simulink model "ThrusterModel0"  (R2018b)
settings: configuration reference "RPi_ControlRate" (kept outside this file)
InitFcn:
  | loadThrusterData
settings Model: Creator=Andy  LastModifiedBy=barthal
settings ConfigSetRef: SourceLocation=Base Workspace

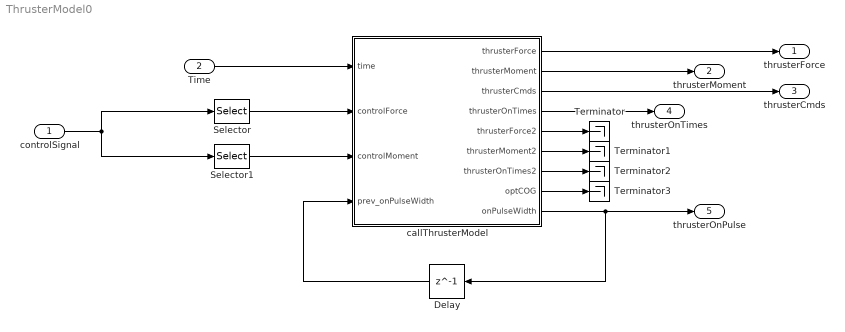
== system ThrusterModel0 ==
  controlSignal : Inport  OutDataTypeStr=double
  Time : Inport  Port=2  OutDataTypeStr=double  PortDimensions=1
  Delay : Delay  DelayLength=1  InitialCondition=[0 0 0 0 0 0 0 0]
  Selector : Selector  InputPortWidth=6  IndexOptions=Index vector (dialog)  Indices=[1 2 3]  OutputSizes=1
  Selector1 : Selector  InputPortWidth=6  IndexOptions=Index vector (dialog)  Indices=[4:6]  OutputSizes=1
  Terminator{,1..3} (4 alike) : Terminator
  callThrusterModel : MATLAB Function  TreatAsAtomicUnit=on
  thrusterForce : Outport  OutDataTypeStr=double
  thrusterMoment : Outport  Port=2  OutDataTypeStr=double
  thrusterCmds : Outport  Port=3  OutDataTypeStr=boolean
  thrusterOnTimes : Outport  Port=4
  thrusterOnPulse : Outport  Port=5
  wires:
  Time/1 -> callThrusterModel/1(time)
  controlSignal/1 -> Selector1/1, Selector/1
  callThrusterModel/4(thrusterOnTimes) -> thrusterOnTimes/1
  callThrusterModel/1(thrusterForce) -> thrusterForce/1
  callThrusterModel/2(thrusterMoment) -> thrusterMoment/1
  Selector/1 -> callThrusterModel/2(controlForce)
  Selector1/1 -> callThrusterModel/3(controlMoment)
  callThrusterModel/3(thrusterCmds) -> thrusterCmds/1
  callThrusterModel/9(onPulseWidth) -> thrusterOnPulse/1, Delay/1
  Delay/1 -> callThrusterModel/4(prev_onPulseWidth)
  callThrusterModel/5(thrusterForce2) -> Terminator/1
  callThrusterModel/6(thrusterMoment2) -> Terminator1/1
  callThrusterModel/7(thrusterOnTimes2) -> Terminator2/1
  callThrusterModel/8(optCOG) -> Terminator3/1

== matlab function ThrusterModel0/callThrusterModel ==
  data: time input; controlForce input; thrusterForce output size=3; controlMoment input; thrusterMoment output size=3; thrusterCmds output; thrusterData parameter; thrusterOnTimes output size=8; thrusterForce2 output size=3; thrusterMoment2 output size=3; thrusterOnTimes2 output size=8; optCOG output size=1; onPulseWidth output; prev_onPulseWidth input
function [thrusterForce,thrusterMoment,thrusterCmds,thrusterOnTimes,thrusterForce2,thrusterMoment2,thrusterOnTimes2,optCOG,onPulseWidth]= callThrusterModel(time,controlForce,controlMoment,thrusterData,prev_onPulseWidth)


[thrusterForce,thrusterMoment,thrusterCmds,thrusterOnTimes,onPulseWidth] = thrusterModel(time,controlForce',controlMoment',thrusterData,prev_onPulseWidth);
[thrusterForce2,thrusterMoment2,thrusterOnTimes2,optCOG] = thrusterModel2(time,controlForce',controlMoment',thrusterData);
